simulink model "MatlabExcavatorModel"  (R2013b)
settings: Solver=FixedStepDiscrete  StartTime=0.0  StopTime=Inf  FixedStep=Auto  RelTol=1e-3
values from neighbouring files (symbols this model uses):
  enginespeed = 2500    [LoadVars.m]
  fuelmatrix = standardfuelmap    [LoadVars.m]
  maxflow_per_rev = 18*cc_2_in3    (= 1.0984273938)    [LoadVars.m]
  maxincol = ones(1,(numengspeeds-1)*engspeeddiv+1)*length(standardtorq)    [fuelmap.m]
  maxpflow = maxflow_per_rev*pumpspeed    [LoadVars.m]
  N2lb = 0.224808943    [LoadVars.m]
  N_m_2_lb_in = 8.85075    [LoadVars.m]
  pheadinit = [tankp tankp tankp tankp]    [LoadVars.m]
  prodinit = [tankp tankp tankp tankp]    [LoadVars.m]
  speedscale = standengspeed    [LoadVars.m]
  torqmax = 170*N_m_2_lb_in    (= 1504.6275)    [LoadVars.m]
  torqscale = newstandardtorq    [LoadVars.m]
  Ts = 0.001    [LoadVars.m]
undefined symbols (not defined in the file): bulkmodulus, fcarm, fcboom, fcbucket, fcswing, fvarm, fvboom, fvbucket, fvswing, KLi_ext_S, leak1, leak2, leak3, leak4, linevol_head1, linevol_head2, linevol_head3, linevol_head4, linevol_rod1, linevol_rod2, linevol_rod3, linevol_rod4, reliefp, tankp
settings Model: ExtModeEnableFloating=off  ExtModeArmWhenConnect=off  Creator=Sam  LastModifiedBy=Sam
settings DataIOCC: LimitDataPoints=off  SaveOutput=off  SignalLogging=off  DSMLogging=off  SaveTime=off
settings OptimizationCC: InlineParams=on  OptimizeModelRefInitCode=on  LifeSpan=Inf
settings DebuggingCC: StateNameClashWarn=warning
settings HardwareCC: ProdHWDeviceType=Generic->Unspecified (assume 32-bit Generic)
settings RTWCC: SystemTargetFile=ert.tlc  TemplateMakefile=RTW.MSVCBuild  Description=Create Visual C/C++ Solution File for the Embedded Coder  ProcessScript=ert_make_rtw_hook  TargetLang=C++  RTWCompilerOptimization=On
settings CodeAppCC: IgnoreTestpoints=on
settings ERTTargetCC: CodeReplacementLibrary=ANSI_C  GenerateSampleERTMain=on  SupportContinuousTime=on  SupportNonInlinedSFcns=on  ERTCustomFileTemplate=example_file_process.tlc

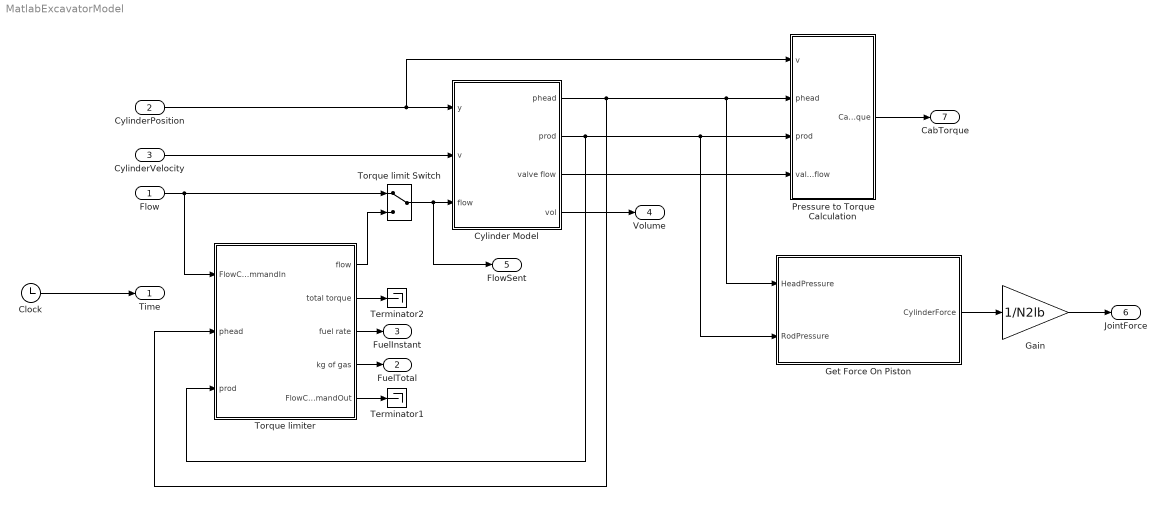
== system MatlabExcavatorModel ==
  "Flow " : Inport  PortDimensions=4
  CylinderPosition : Inport  Port=2  PortDimensions=4
  CylinderVelocity : Inport  Port=3
  Clock : Clock
  Cylinder Model : Subsystem  mask{Ts=Ts, ptank=tankp, bulk_mod=bulkmodulus, lvolh1=linevol_head1, lvolh2=linevol_head2, lvolh3=linevol_head3, lvolh4=linevol_head4, lvolr1=linevol_rod1, lvolr2=linevol_rod2, lvolr3=linevol_rod3, lvolr4=linevol_rod4, head1=4, head2=4, head3=4, head4=4, rod1=5, rod2=5, rod3=5, rod4=5, prelief1=reliefp, prelief2=reliefp, prelief3=reliefp, prelief4=reliefp, leak1=(leak1 + KLi_ext_S), leak2=leak2, leak3=leak3, leak4=leak4}
      mask prompts: Ts "Sampling Time (s)"; ptank "Tank pressure (psi)"; bulk_mod "Effective fluid bulk modulus (psi)"; lvolh1 "Line volume on the head side for the swing (in^3)"; lvolh2 "Line volume on the head side for the boom (in^3)"; lvolh3 "Line volume on the head side for the arm (in^3)"; lvolh4 "Line volume on the head side for the bucket (in^3)"; lvolr1 "Line volume on the rod side for the swing (in^3)"; lvolr2 "Line volume on the rod side for the boom (in^3)"; lvolr3 "Line volume on the rod side for the arm (in^3)"; lvolr4 "Line volume on the rod side for the bucket (in^3)"; head1 "Swing head length (in) (unused)"; head2 "Boom head length (in)"; head3 "Arm head length (in)"; head4 "Bucket head length (in)"; rod1 "Rod end length for swing (in) (unused)"; rod2 "Rod end length for boom (in)"; rod3 "Rod end length for arm (in)"; rod4 "Rod end length for bucket (in)"; prelief1 "Relief valve pressure for swing (psi)"; prelief2 "Relief valve pressure for boom (psi)"; prelief3 "Relief valve pressure for arm (psi)"; prelief4 "Relief valve pressure for bucket (psi)"; leak1 "Leakage coeff for swing (in^3/s/psi)"; leak2 "Leakage coeff for boom (in^3/s/psi)"; leak3 "Leakage coeff for arm (in^3/s/psi)"; leak4 "Leakage coeff for bucket (in^3/s/psi)"
  Gain : Gain  Gain=1/N2lb
  Get Force On Piston : MATLAB Function  TreatAsAtomicUnit=on
  Pressure to Torque Calculation : Subsystem  mask{Ts=Ts, fv_swing=fvswing, fv_boom=fvboom, fv_arm=fvarm, fv_bucket=fvbucket, fc_swing=fcswing, fc_boom=fcboom, fc_arm=fcarm, fc_bucket=fcbucket, fbrake=50000}
      mask prompts: Ts "Sampling time (sec)"; fv_swing "Swing Viscous Frictional Coeff (Ft lb s)"; fv_boom "Boom Viscous Frictional Coeff (kg/s)"; fv_arm "Arm Viscous Frictional Coeff (kg/s)"; fv_bucket "Bucket Viscous Frictional Coeff (kg/s)"; fc_swing "Swing Coulombic Frictional Coeff"; fc_boom "Boom Coulombic Frictional Coeff"; fc_arm "Arm Coulombic Frictional Coeff"; fc_bucket "Bucket Coulombic Frictional Coeff"; fbrake "Valve Braking Coeff"
  Terminator1 : Terminator
  Terminator2 : Terminator
  Torque limit Switch : ManualSwitch
  Torque limiter : Subsystem
  Time : Outport
  FuelTotal : Outport  Port=2
  FuelInstant : Outport  Port=3
  "Volume " : Outport  Port=4
  FlowSent : Outport  Port=5
  JointForce : Outport  Port=6
  CabTorque : Outport  Port=7  PortDimensions=1
  wires:
  CylinderPosition/1 -> Cylinder Model/1(y), Pressure to Torque Calculation/1(v)
  CylinderVelocity/1 -> Cylinder Model/2(v)
  Cylinder Model/4(vol) -> "Volume "/1
  Torque limit Switch/1 -> FlowSent/1, Cylinder Model/3(flow)
  Torque limiter/4(kg of gas) -> FuelTotal/1
  Torque limiter/3(fuel rate) -> FuelInstant/1
  Clock/1 -> Time/1
  Torque limiter/2(total torque) -> Terminator2/1
  Torque limiter/1(flow) -> Torque limit Switch/2
  Cylinder Model/2(prod) -> Get Force On Piston/2(RodPressure), Pressure to Torque Calculation/3(prod), Torque limiter/3(prod)
  Cylinder Model/1(phead) -> Torque limiter/2(phead), Pressure to Torque Calculation/2(phead), Get Force On Piston/1(HeadPressure)
  Torque limiter/5(FlowCommandOut) -> Terminator1/1
  "Flow "/1 -> Torque limiter/1(FlowCommandIn), Torque limit Switch/1
  Cylinder Model/3(valve flow) -> Pressure to Torque Calculation/4(valve flow)
  Get Force On Piston/1(CylinderForce) -> Gain/1
  Gain/1 -> JointForce/1
  Pressure to Torque Calculation/1(CabTorque) -> CabTorque/1

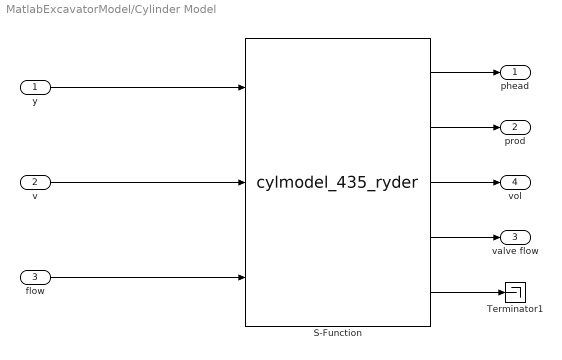
== system MatlabExcavatorModel/Cylinder Model ==
  y : Inport
  v : Inport  Port=2
  flow : Inport  Port=3
  S-Function : S-Function  FunctionName=cylmodel_435_ryder  Parameters=Ts, ptank, bulk_mod, lvolh1, lvolh2, lvolh3, lvolh4, lvolr1, lvolr2, lvolr3, lvolr4, head1, head2, head3, head4, rod1, rod2, rod3, rod4, prelief1, prelief2, prelief3, prelief4, leak1, leak2, leak3, leak4  EnableBusSupport=off
  Terminator1 : Terminator
  phead : Outport
  prod : Outport  Port=2
  valve flow : Outport  Port=3
  vol : Outport  Port=4
  wires:
  y/1 -> S-Function/1
  S-Function/1 -> phead/1
  v/1 -> S-Function/2
  S-Function/2 -> prod/1
  flow/1 -> S-Function/3
  S-Function/3 -> vol/1
  S-Function/4 -> valve flow/1
  S-Function/5 -> Terminator1/1

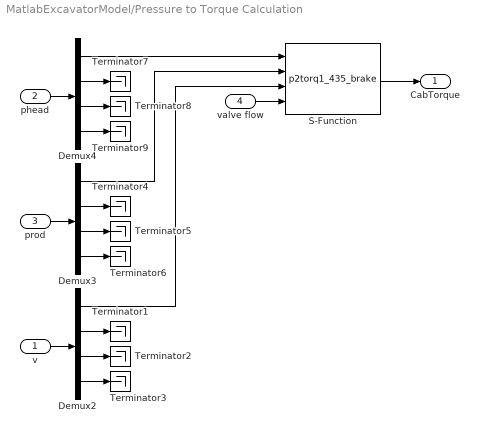
== system MatlabExcavatorModel/Pressure to Torque Calculation ==
  v : Inport
  phead : Inport  Port=2
  prod : Inport  Port=3
  valve flow : Inport  Port=4
  Demux2 : Demux
  Demux3 : Demux
  Demux4 : Demux
  S-Function : S-Function  FunctionName=p2torq1_435_brake  Parameters=Ts, fv_swing, fc_swing, fbrake  EnableBusSupport=off
  Terminator{1..9} (9 alike) : Terminator
  CabTorque : Outport  PortDimensions=1
  wires:
  Demux4/1 -> S-Function/1
  Demux3/1 -> S-Function/2
  Demux2/1 -> S-Function/3
  Demux2/2 -> Terminator1/1
  v/1 -> Demux2/1
  valve flow/1 -> S-Function/4
  S-Function/1 -> CabTorque/1
  Demux2/3 -> Terminator2/1
  Demux2/4 -> Terminator3/1
  Demux3/2 -> Terminator4/1
  prod/1 -> Demux3/1
  Demux3/3 -> Terminator5/1
  Demux3/4 -> Terminator6/1
  Demux4/2 -> Terminator7/1
  phead/1 -> Demux4/1
  Demux4/3 -> Terminator8/1
  Demux4/4 -> Terminator9/1

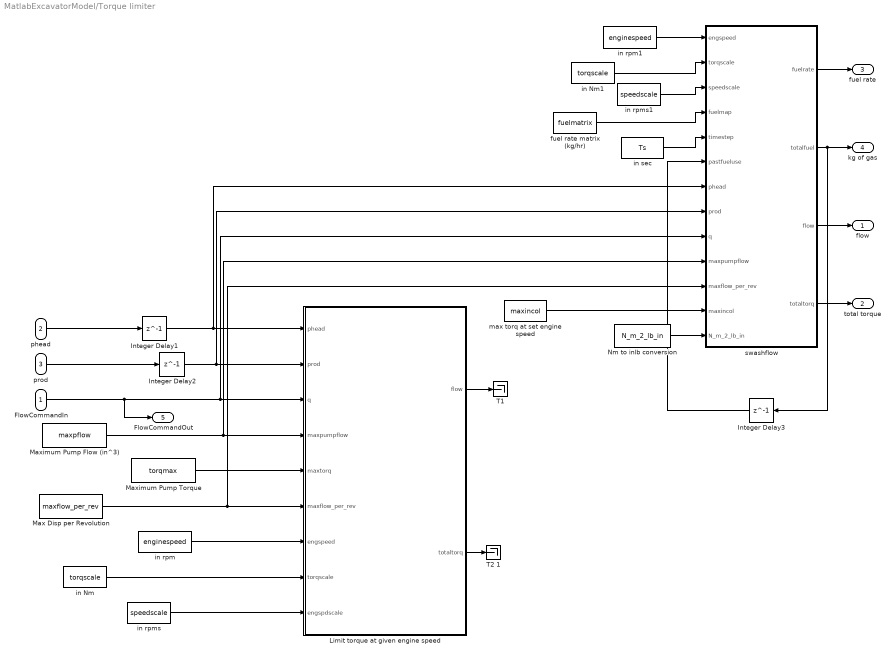
== system MatlabExcavatorModel/Torque limiter ==
  FlowCommandIn : Inport
  phead : Inport  Port=2
  prod : Inport  Port=3
  Integer Delay1 : Delay  DelayLength=1  InitialCondition=pheadinit  InputProcessing=Inherited
  Integer Delay2 : Delay  DelayLength=1  InitialCondition=prodinit  InputProcessing=Inherited
  Integer Delay3 : Delay  DelayLength=1  InitialCondition=0  InputProcessing=Inherited
  Limit torque at given engine speed : MATLAB Function  TreatAsAtomicUnit=on
  Max Disp per Revolution : Constant  Value=maxflow_per_rev  VectorParams1D=off
  Maximum Pump Flow (in^3) : Constant  Value=maxpflow  VectorParams1D=off
  Maximum Pump Torque : Constant  Value=torqmax  VectorParams1D=off
  Nm to inlb conversion : Constant  Value=N_m_2_lb_in
  "T1 " : Terminator
  T2 1 : Terminator
  fuel rate matrix (kg/hr) : Constant  Value=fuelmatrix  VectorParams1D=off
  in Nm : Constant  Value=torqscale
  in Nm1 : Constant  Value=torqscale
  in rpm : Constant  Value=enginespeed
  in rpm1 : Constant  Value=enginespeed
  in rpms : Constant  Value=speedscale
  in rpms1 : Constant  Value=speedscale
  in sec : Constant  Value=Ts
  max torq at set engine speed : Constant  Value=maxincol
  swashflow : MATLAB Function  TreatAsAtomicUnit=on
  flow : Outport
  total torque : Outport  Port=2
  fuel rate : Outport  Port=3
  kg of gas : Outport  Port=4
  FlowCommandOut : Outport  Port=5
  wires:
  prod/1 -> Integer Delay2/1
  Integer Delay2/1 -> Limit torque at given engine speed/2(prod), swashflow/8(prod)
  Maximum Pump Flow (in^3)/1 -> Limit torque at given engine speed/4(maxpumpflow), swashflow/10(maxpumpflow)
  Maximum Pump Torque/1 -> Limit torque at given engine speed/5(maxtorq)
  Max Disp per Revolution/1 -> Limit torque at given engine speed/6(maxflow_per_rev), swashflow/11(maxflow_per_rev)
  FlowCommandIn/1 -> FlowCommandOut/1, Limit torque at given engine speed/3(q), swashflow/9(q)
  Integer Delay1/1 -> Limit torque at given engine speed/1(phead), swashflow/7(phead)
  phead/1 -> Integer Delay1/1
  in rpm/1 -> Limit torque at given engine speed/7(engspeed)
  in Nm/1 -> Limit torque at given engine speed/8(torqscale)
  in rpms/1 -> Limit torque at given engine speed/9(engspdscale)
  in rpm1/1 -> swashflow/1(engspeed)
  in Nm1/1 -> swashflow/2(torqscale)
  in rpms1/1 -> swashflow/3(speedscale)
  fuel rate matrix (kg/hr)/1 -> swashflow/4(fuelmap)
  swashflow/1(fuelrate) -> fuel rate/1
  swashflow/2(totalfuel) -> kg of gas/1, Integer Delay3/1
  in sec/1 -> swashflow/5(timestep)
  Integer Delay3/1 -> swashflow/6(pastfueluse)
  swashflow/3(flow) -> flow/1
  swashflow/4(totaltorq) -> total torque/1
  max torq at set engine speed/1 -> swashflow/12(maxincol)
  Nm to inlb conversion/1 -> swashflow/13(N_m_2_lb_in)
  Limit torque at given engine speed/1(flow) -> "T1 "/1
  Limit torque at given engine speed/2(totaltorq) -> T2 1/1

== matlab function MatlabExcavatorModel/Get Force On Piston ==
  data: CylinderForce output; HeadPressure input; RodPressure input
% This function reads in swashplate data and interpolates and then calculates the flow

function CylinderForce   = ForceCalc(HeadPressure, RodPressure)
boreDiameters = [0; 3.75; 3.25; 3.0];
rodDiameters = [0; 2; 2; 1.75];
boreRadius = boreDiameters/2;
rodRadius = rodDiameters/2;
headArea = boreRadius .* boreRadius * pi;
rodArea = headArea - (rodRadius .* rodRadius * pi);
CylinderForce = HeadPressure .* headArea - RodPressure .* rodArea;
CylinderForce = CylinderForce;

== matlab function MatlabExcavatorModel/Torque limiter/swashflow ==
  data: fuelrate output; engspeed input; torqscale input; speedscale input; fuelmap input; timestep input; pastfueluse input; totalfuel output; phead input; prod input; q input; maxpumpflow input; maxflow_per_rev input; flow output; totaltorq output; maxincol input; N_m_2_lb_in input
% This function reads in swashplate data and interpolates and then calculates the flow
%function [flow, totaltorq] = torq_limited( maxtorq, )
function [fuelrate, totalfuel, flow, totaltorq]  = fuelusage(engspeed,torqscale,speedscale,...
    fuelmap,timestep,pastfueluse,phead, prod, q, maxpumpflow,maxflow_per_rev, maxincol, N_m_2_lb_in)

d_engspd = speedscale(2)-speedscale(1);
d_torq = torqscale(2)-torqscale(1);

if (engspeed <= speedscale(1))
    spdindex = 1;
else
    if (engspeed >= speedscale(length(speedscale)))
        spdindex = length(speedscale);
    else
        spdindex = floor( (engspeed-speedscale(1))/d_engspd ) + 1;
    end
end

flowout = q;
flowpercent = zeros(1,4);
flowperrev = zeros(1,4);
for k = 1:4
    flowpercent(k) = q(k)/maxpumpflow(k);
    flowperrev(k) = flowpercent(k)*maxflow_per_rev;
end
% calculate needed torq for current demand
totaltorq = 0;
for k=1:4
    totaltorq = totaltorq + (phead(k)-prod(k))*flowperrev(k)/(2*pi);%.001/8.851;
end
maxtorq = torqscale(maxincol(spdindex));

if (totaltorq > maxtorq)%( isnan(fuelmap(spdindex,torqindex)) ) % need to limit torque
    %torqindex = maxincol(spdindex);
    %torq = torqscale(torqindex);

    % calculate % reduction rate based on torque limit
    %if (totaltorq > maxtorq)
        torq_reduce = totaltorq/maxtorq;
    %else
     %   torq_reduce = 1;
    %end

    % reduce flow evenly for all cylinders
    for k = 1:4
        %flowout(k) = q(k)/hp_reduce;
        flowout(k) = q(k)/torq_reduce;
    end
end
% calculate limited torque (to check that it's < max torque)
totaltorq = 0;
for k = 1:4
    flowpercent(k) = flowout(k)/maxpumpflow(k);
    flowperrev(k) = flowpercent(k)*maxflow_per_rev;
    totaltorq = totaltorq + (phead(k)-prod(k))*flowperrev(k)/(2*pi);
end

flow = flowout .* [1; 1; 1; 1];

torq = totaltorq/N_m_2_lb_in;

if (torq <= 0 )
   torq = 0;
end
if (torq <= torqscale(1))
    torqindex = 1;
else
    if (torq >= torqscale(length(torqscale)))
        torqindex = length(torqscale);
    else
        torqindex = floor( (torq-torqscale(1))/d_torq ) + 1;
    end
end

if ( isnan(fuelmap(spdindex+1,torqindex)) )
    spdslope = (fuelmap(spdindex,torqindex) - fuelmap(spdindex-1,torqindex))/d_engspd;
else
    spdslope = (fuelmap(spdindex+1,torqindex) - fuelmap(spdindex,torqindex))/d_engspd;
end

if ( isnan(fuelmap(spdindex,torqindex+1)) )
    torqslope = (fuelmap(spdindex,torqindex)- fuelmap(spdindex,torqindex-1))/d_torq;
else
    torqslope = (fuelmap(spdindex,torqindex+1)- fuelmap(spdindex,torqindex))/d_torq;
end

spdincrease = spdslope * (engspeed - speedscale(spdindex));
torqincrease = torqslope * (torq - torqscale(torqindex));

fuelrate = fuelmap(spdindex,torqindex) + spdincrease + torqincrease;

totalfuel = pastfueluse + fuelrate*timestep/3600;

== matlab function MatlabExcavatorModel/Torque limiter/Limit torque at given engine speed ==
  data: phead input; flow output; prod input; q input; totaltorq output; maxpumpflow input; maxtorq input; maxflow_per_rev input; engspeed input; torqscale input; engspdscale input
% this function limits the pump output evenly for all 4 pumps when the
% maximum allowable torque is exceeded

% phead is head side pressure in psi
% prod is rod side pressure in psi
% q is flow in in^3/sec
% maxpumpflow is the max displacement of the pumps being driven at pumpspeed
% maxtorq is the max torque rating of the diesel engine in inch lbs
% maxflow_per_rev is the full displacement of the pump in in^3/rev

function [flow, totaltorq] = torq_limited(phead, prod, q, maxpumpflow, maxtorq, maxflow_per_rev,engspeed,torqscale,engspdscale)

flowout = zeros(1,4);
flowpercent = zeros(1,4);
flowperrev = zeros(1,4);
% maxhp = 49;

for k = 1:4
    flowpercent(k) = q(k)/maxpumpflow(k);
    flowperrev(k) = flowpercent(k)*maxflow_per_rev;
end

% calculate needed torq for current demand
totaltorq = 0;
for k=1:4
    totaltorq = totaltorq + (phead(k)-prod(k))*flowperrev(k)/(2*pi);%.001/8.851;
end

% calculate % reduction rate based on torque limit
if (totaltorq > maxtorq)
    torq_reduce = totaltorq/maxtorq;
else
    torq_reduce = 1;
end

% % calculate needed hp for current demand
% totalhp = 0;
% for k=1:4
%     totalhp = totalhp + (phead(k)-prod(k))*q(k)/12/550;
% end
% 
% % calculate % reduction rate off hp limit
% if (totalhp > maxhp)
%     hp_reduce = totalhp/maxhp;
% else
%     hp_reduce = 1;
% end

% reduce flow evenly for all cylinders
for k = 1:4
    %flowout(k) = q(k)/hp_reduce;
    flowout(k) = q(k)/torq_reduce;
end

% % calculate limited hp (to check that it's < max hp)
% totalhp = 0;
% for k = 1:4
%     totalhp = totalhp + (phead(k)-prod(k))*flowout(k)/12/550;
% end

% calculate limited torque (to check that it's < max torque)
totaltorq = 0;
for k = 1:4
    flowpercent(k) = flowout(k)/maxpumpflow(k);
    flowperrev(k) = flowpercent(k)*maxflow_per_rev;
    totaltorq = totaltorq + (phead(k)-prod(k))*flowperrev(k)/(2*pi);
end

flow = flowout';
